simulink model "Forward_Kinmeatics"  (R2022b)
settings: Solver=VariableStepAuto  StartTime=0.0  StopTime=10.0  RelTol=1e-3
settings Model: Creator=sathwik  LastModifiedBy=sathwik

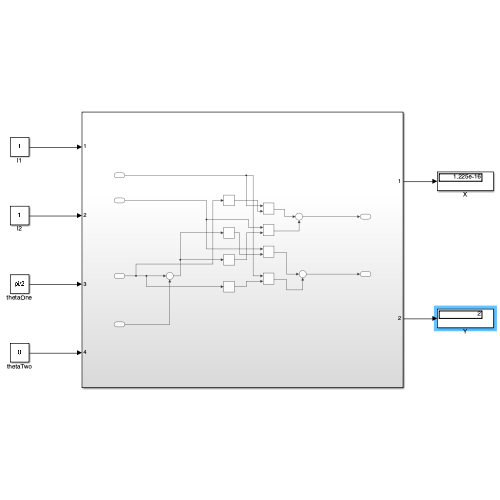
[thumbnail: Simulink's stored preview of the top-level diagram]
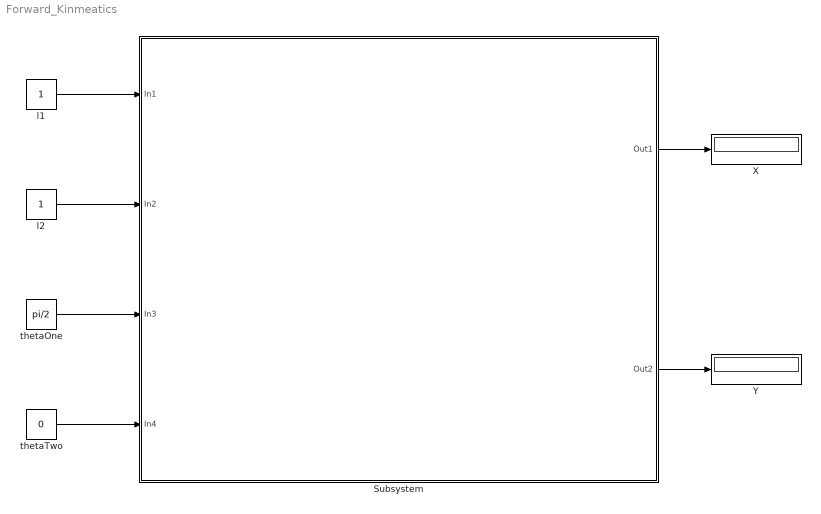
== system Forward_Kinmeatics ==
  Subsystem : Subsystem
  X : Display
  Y : Display
  l1 : Constant
  l2 : Constant
  thetaOne : Constant  Value=pi/2
  thetaTwo : Constant  Value=0
  wires:
  l1/1 -> Subsystem/1(In1)
  l2/1 -> Subsystem/2(In2)
  thetaOne/1 -> Subsystem/3(In3)
  thetaTwo/1 -> Subsystem/4(In4)
  Subsystem/1(Out1) -> X/1
  Subsystem/2(Out2) -> Y/1

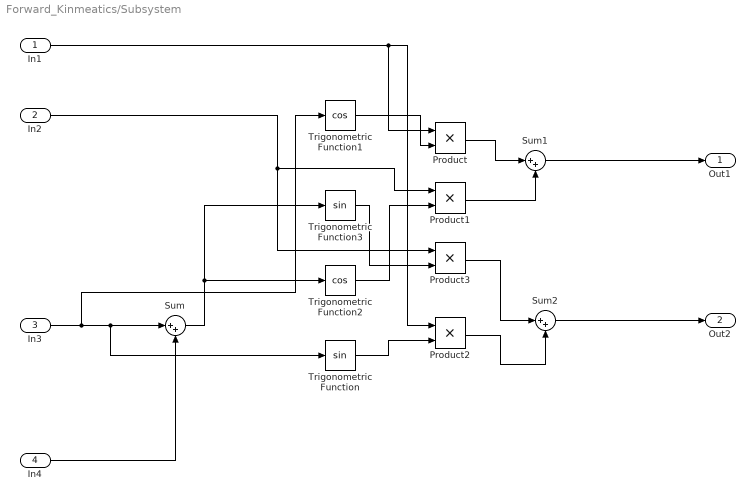
== system Forward_Kinmeatics/Subsystem ==
  In1 : Inport
  In2 : Inport  Port=2
  In3 : Inport  Port=3
  In4 : Inport  Port=4
  Product{,1..3} (4 alike) : Product
  Sum : Sum  Inputs=|++
  Sum1 : Sum  Inputs=|++
  Sum2 : Sum  Inputs=|++
  Trigonometric Function : Trigonometry
  Trigonometric Function1 : Trigonometry  Operator=cos
  Trigonometric Function2 : Trigonometry  Operator=cos
  Trigonometric Function3 : Trigonometry
  Out1 : Outport
  Out2 : Outport  Port=2
  wires:
  Sum2/1 -> Out2/1
  In4/1 -> Sum/2
  Sum1/1 -> Out1/1
  Product3/1 -> Sum2/1
  In1/1 -> Product2/1, Product/1
  Product/1 -> Sum1/1
  Product1/1 -> Sum1/2
  Trigonometric Function1/1 -> Product/2
  Sum/1 -> Trigonometric Function3/1, Trigonometric Function2/1
  Product2/1 -> Sum2/2
  In2/1 -> Product3/1, Product1/1
  Trigonometric Function2/1 -> Product1/2
  Trigonometric Function3/1 -> Product3/2
  In3/1 -> Trigonometric Function1/1, Trigonometric Function/1, Sum/1
  Trigonometric Function/1 -> Product2/2
